simulink model "Dan_model3a"  (Simulink 7.8)
settings: Solver=ode45  StartTime=0.0  StopTime=10.0  RelTol=1e-3
values from neighbouring files (symbols this model uses):
  h = h_vec(i)    [ps7-task3.m]
libraries: cstblocks x2
settings Model: Creator=lifeofsacrifice  LastModifiedBy=Dan
settings DebuggingCC: InitInArrayFormatMsg=none

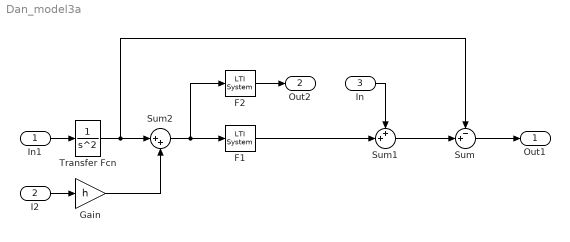
== system Dan_model3a ==
  In1 : Inport
  I2 : Inport  Port=2
  In : Inport  Port=3
  F1 : cstblocks/LTI System  sys=F1  IC=[]
  F2 : cstblocks/LTI System  sys=F2  IC=[]
  Gain : Gain  Gain=h
  Sum : Sum  Inputs=-+|
  Sum1 : Sum  Inputs=++|
  Sum2 : Sum  Inputs=|++
  Transfer Fcn : TransferFcn  Denominator=[1 0 0]
  Out1 : Outport
  Out2 : Outport  Port=2
  wires:
  In1/1 -> Transfer Fcn/1
  Transfer Fcn/1 -> Sum2/1, Sum/1
  I2/1 -> Gain/1
  Gain/1 -> Sum2/2
  Sum2/1 -> F2/1, F1/1
  Sum/1 -> Out1/1
  F2/1 -> Out2/1
  Sum1/1 -> Sum/2
  In/1 -> Sum1/1
  F1/1 -> Sum1/2
